simulink model "car_model_FIXED"  (R2022b)
settings: Solver=VariableStepAuto  StartTime=0.0  StopTime=60  RelTol=1e-3
values from neighbouring files (symbols this model uses):
  ABS_MAX_TORQUE = [25 25 25 25]    [workspace.mat]
  ABS_MAX_TRQ_CMD = 50    [workspace.mat]
  ABS_MIN_TORQUE = [0.01 0.01 0.01 0.01]    [workspace.mat]
  acc_IC = 0    [workspace.mat]
  ACCELERATION_MAX = 30    [workspace.mat]
  ActSuspDutyCycle = 1    [workspace.mat]
  Aeq_left = [0.305756190204 0.308857786592 0.311945941182 0.315020811431 0.318082554689 0.321131328186 0.324167289011 0.327190594103 0.330201400225 0.333199863958 0.336186141681 0.339160389558 ... (261 elements, 1x261)]    [workspace.mat]
  Aeq_right = [-0.961664782545 -0.959835898365 -0.957982924115 -0.956106413788 -0.954206913862 -0.952284963337 -0.950341093764 -0.948375829284 -0.946389686656 -0.944383175301 -0.942356797333 -0.940311047601 ... (261 elements, 1x261)]    [workspace.mat]
  alpha_error = 0.1    [workspace.mat]
  ang_acc_hystersesis = 0.1    [workspace.mat]
  ang_IC = 0    [workspace.mat]
  ang_vel_IC = 0    [workspace.mat]
  area_air = 0.15    [workspace.mat]
  axb = -5    [workspace.mat]
  battery_current_IC = 0    [workspace.mat]
  BATTERY_CURRENT_MAX = 140    [workspace.mat]
  BATTERY_CURRENT_MIN = 0    [workspace.mat]
  battery_FT_IC = 300    [workspace.mat]
  battery_T_IC = 300    [workspace.mat]
  BATTERY_TEMPERATURE_MAX = 60    [workspace.mat]
  BATTERY_TEMPERATURE_MIN = 0    [workspace.mat]
  battery_voltage_IC = 332    [workspace.mat]
  BATTERY_VOLTAGE_MAX = 340    [workspace.mat]
  BATTERY_VOLTAGE_MIN = 60    [workspace.mat]
  br = 0.01    [workspace.mat]
  brake_bias = [0.35 0.35 0.15 0.15]    [workspace.mat]
  Brake_Pressure_IC = 1    [workspace.mat]
  ccl_IC = 0    [workspace.mat]
  CENTER_STEER_ANGLE_MAX = 130    [workspace.mat]
  covarience_matrix_IC = [0.001 0 0 0 0 0 0 0 0 0 0 0 ... (784 elements, 28x28)]    [workspace.mat]
  CURRENT_BUFFER = 25    [workspace.mat]
  cy_sweep = [13568.4166816 14020.2069783 14456.754831 14879.7402576 15289.7264712 15687.2766846 16072.954111 16447.3219632 16810.9434544 17164.3817975 17508.2002054 17842.9618912 ... (101 elements, 1x101)]    [workspace.mat]
  dB = 0.001    [workspace.mat]
  dcl_IC = 140    [workspace.mat]
  DCL_MAX = 130    [workspace.mat]
  DCL_MIN = 0    [workspace.mat]
  deadband_angle = 12    [workspace.mat]
  dIndex = 50    [workspace.mat]
  driver_t = 0.015    [workspace.mat]
  dt_OFF = 4.5    [workspace.mat]
  dt_ON = 7.5    [workspace.mat]
  dTx = 0.01    [workspace.mat]
  dx = 0.1    [workspace.mat]
  dZ = 0.295    [workspace.mat]
  efficiency_grid = [0.759500051293 0.787587791453 0.809832189108 0.826747821898 0.837164543102 0.842744381136 0.842258400104 0.838611650621 0.82826195101 0.814029316176 0.795690627225 0.7759791486 ... (2782 elements, 26x107)]    [workspace.mat]
  F0z = [0 0]    [workspace.mat]
  forward_look_straight = 5    [workspace.mat]
  forward_look_turn = 15    [workspace.mat]
  Fz_IC = 539.55    [workspace.mat]
  Fz_sweep = [200 210 220 230 240 250 260 270 280 290 300 310 ... (101 elements, 1x101)]    [workspace.mat]
  g = 9.81    [workspace.mat]
  GAIN_ABS = 100    [workspace.mat]
  gearbox_efficiency = [0.8 0.8 0.8 0.8]    [workspace.mat]
  gps_counter_IC = 0    [workspace.mat]
  gps_hz = 0.01    [workspace.mat]
  gr = [8.74786324786 8.74786324786 8.74786324786 8.74786324786]    [workspace.mat]
  I = 0    [workspace.mat]
  I_Driver = 1    [workspace.mat]
  indicies = [3 3.5 4 0.5 1 1.5 2 2.5 3 3.5 4 0.5 ... (27 elements, 1x27)]    [workspace.mat]
  IYY = 0.3    [workspace.mat]
  kx_sweep = [8779.958 9178.302 9576.646 9974.99 10373.334 10771.678 11170.022 11568.366 11966.71 12365.054 12763.398 13161.742 ... (101 elements, 1x101)]    [workspace.mat]
  l = [0.772 0.772]    [workspace.mat]
  lambda_star = 0.15    [workspace.mat]
  low_V_SA = 0.001    [workspace.mat]
  lr = 35    [workspace.mat]
  m_all = 220    [workspace.mat]
  m_body = 180    [workspace.mat]
  m_unsprung = [6 6 14 14]    [workspace.mat]
  MAG_MAX = 200    [workspace.mat]
  Max_Brake_Pressure = 100000000    [workspace.mat]
  Max_Driver_Input = 1    [workspace.mat]
  MAX_DTHETA_DRIVER = 360    [workspace.mat]
  MAX_I_Driver = 1    [workspace.mat]
  MAX_STEERING_ADJUST = 15    [workspace.mat]
  max_yaw = [0.705271610162 0.928228152446 1.12280857731 1.14131008363 1.08727026041 1.01377803859 0.938114723816 0.8718206875 0.815009168116 0.767481919497 0.727119764215 0.694403589394 ... (15 elements, 1x15)]    [workspace.mat]
  Min_Brake_Pressure = 1    [workspace.mat]
  Min_Driver_Input = 0    [workspace.mat]
  min_velocity_regen = 1.4    [workspace.mat]
  motor_current_IC = 0    [workspace.mat]
  MOTOR_CURRENT_MAX = 70    [workspace.mat]
  MOTOR_CURRENT_MIN = 0    [workspace.mat]
  MOTOR_ENABLE = [0 0 1 1]    [workspace.mat]
  motor_FT_IC = 300    [workspace.mat]
  motor_T_IC = 300    [workspace.mat]
  MOTOR_TEMPERATURE_MAX = 100    [workspace.mat]
  MOTOR_TEMPERATURE_MIN = 0    [workspace.mat]
  motor_voltage_IC = 332    [workspace.mat]
  MOTOR_VOLTAGE_MAX = 340    [workspace.mat]
  MOTOR_VOLTAGE_MIN = 90    [workspace.mat]
  motorControllerCurve = [25  260; 50  130; 75  0]    [workspace.mat]
  motorTempCurve = [140 138.6 134.4 127.4 117.6 105 89.6 71.4 50.4 26.6 0]    [workspace.mat]
  motorTempX = [75 77 79 81 83 85 87 89 91 93 95]    [workspace.mat]
  mu_star = 0.5    [workspace.mat]
  mx_sweep = [3.38348 3.3655067 3.3477908 3.3303323 3.3131312 3.2961875 3.2795012 3.2630723 3.2469008 3.2309867 3.21533 3.1999307 ... (101 elements, 1x101)]    [workspace.mat]
  my_sweep = [3.036232 3.015241699 2.994987032 2.975452753 2.956623616 2.938484375 2.921019784 2.904214597 2.888053568 2.872521451 2.857603 2.843282969 ... (101 elements, 1x101)]    [workspace.mat]
  noise_state = [1e-06 1e-06 1e-06 1e-06 0.005 0.005 0.005 1e-06 1e-06 1e-06 1e-06 1e-06 ... (28 elements, 28x1)]    [workspace.mat]
  omega_IC = 0    [workspace.mat]
  OMEGA_MAX = 150    [workspace.mat]
  OMEGA_MIN = 0    [workspace.mat]
  ORIENTATION_MAX = 360    [workspace.mat]
  P = 2    [workspace.mat]
  P_Driver = 0.7    [workspace.mat]
  P_High_Speed = 0.1    [workspace.mat]
  P_Steering_Adjust = 2    [workspace.mat]
  P_Straight_Adjust = 5    [workspace.mat]
  pos_IC = 0    [workspace.mat]
  POS_MAX = 300    [workspace.mat]
  q_thresh = 0.3    [workspace.mat]
  RE = 0.223    [workspace.mat]
  rho = 1.225    [workspace.mat]
  s = [0.649 0.621]    [workspace.mat]
  selected_maxvm = [49.86390724 16.21289794 8.219813569 8.05215527 7.103352929 8.35634983 13.87515039 8.72402841 22.75224945 36.67909339 19.32001297 25.09036962 ... (63 elements, 21x3)]    [workspace.mat]
  selected_sweep = [3 3 3 3 3 3 3 3 3 3 3 3 ... (1288 elements, 644x2)]    [workspace.mat]
  selected_track = [inf inf inf inf inf inf inf inf inf inf inf inf ... (37971 elements, 4219x9)]    [workspace.mat]
  shock_length_IC = 0.1    [workspace.mat]
  SHOCK_LENGTH_MAX = 0.25    [workspace.mat]
  SHOCK_LENGTH_MIN = 0    [workspace.mat]
  state_IC = [1 0 0 0 0 0 0 0 0 0 0 0 ... (28 elements, 28x1)]    [workspace.mat]
  steering_sweep = [0 5 10 15 20 25 30 35 40 45 50 55 ... (27 elements, 1x27)]    [workspace.mat]
  steering_Up_Grid = [0.551231966244 8.36038106007 16.1333806643 23.9559539118 31.8240691982 39.7561724339 47.7157531433 55.7845698794 64.1341708168 73.0798046026 82.7903081349 93.1297322155 ... (615 elements, 41x15)]    [workspace.mat]
  ... (+25 more)
undefined symbols (not defined in the file or in its folder): ax, ay, az, covA, covG, covM, covP, covV, DiscIntNeverNeededParam, fusion_t, fusion_t_sim, gps_ratio, IMU_accel, IMU_gyro, imu_hz, IMU_mag, location_lla_IC, p, phi, psi, q, r, sus, theta, trn, veh, VEH, whl, X, Xdot, Y, Ydot, Z, Zdot
libraries: fl_lib x82, nesl_utility x32, vehdynlibtire x10, vehdynlibsuspension x8, simulink x5, autolibutils x5, sharedtransform x5, sdl_lib x4, EngineCoolingComponents_lib x4, slpidlib x3, SimscapeFluids_lib x3, shared6dof x2
(part 14 of 14)

== system car_model_FIXED/Vehicle Model/Wheels and Tires/VDBS/Tires/Fiala Tires/z ==
  In1 : Inport
  In2 : Inport  Port=2
  In3 : Inport  Port=3
  In4 : Inport  Port=4
  Bus Selector{,1..3} (4 alike) : BusSelector  OutputSignals=z
  Vector Concatenate : Concatenate  NumInputs=4
  Out1 : Outport  VectorParamsAs1DForOutWhenUnconnected=off
  wires:
  Bus Selector3/1 -> Vector Concatenate/4  "<z>"
  Bus Selector2/1 -> Vector Concatenate/3  "<z>"
  Bus Selector1/1 -> Vector Concatenate/2  "<z>"
  In4/1 -> Bus Selector3/1
  In3/1 -> Bus Selector2/1
  In2/1 -> Bus Selector1/1
  Bus Selector/1 -> Vector Concatenate/1  "<z>"
  In1/1 -> Bus Selector/1
  Vector Concatenate/1 -> Out1/1

== system car_model_FIXED/Vehicle Model/Wheels and Tires/VDBS/Tires/Fiala Tires/zdot ==
  In1 : Inport
  In2 : Inport  Port=2
  In3 : Inport  Port=3
  In4 : Inport  Port=4
  Bus Selector{,1..3} (4 alike) : BusSelector  OutputSignals=zdot
  Vector Concatenate : Concatenate  NumInputs=4
  Out1 : Outport  VectorParamsAs1DForOutWhenUnconnected=off
  wires:
  Vector Concatenate/1 -> Out1/1
  In1/1 -> Bus Selector/1
  Bus Selector/1 -> Vector Concatenate/1  "<zdot>"
  In2/1 -> Bus Selector1/1
  In3/1 -> Bus Selector2/1
  In4/1 -> Bus Selector3/1
  Bus Selector1/1 -> Vector Concatenate/2  "<zdot>"
  Bus Selector2/1 -> Vector Concatenate/3  "<zdot>"
  Bus Selector3/1 -> Vector Concatenate/4  "<zdot>"

== system car_model_FIXED/Vehicle Model/Wheels and Tires/VDBS/Tires/MF Tires/Fx ==
  In1 : Inport
  In2 : Inport  Port=2
  In3 : Inport  Port=3
  In4 : Inport  Port=4
  Bus Selector{,1..3} (4 alike) : BusSelector  OutputSignals=Fx
  Vector Concatenate : Concatenate  NumInputs=4
  Out1 : Outport  VectorParamsAs1DForOutWhenUnconnected=off
  wires:
  Bus Selector3/1 -> Vector Concatenate/4  "<Fx>"
  Bus Selector2/1 -> Vector Concatenate/3  "<Fx>"
  Bus Selector1/1 -> Vector Concatenate/2  "<Fx>"
  In4/1 -> Bus Selector3/1
  In3/1 -> Bus Selector2/1
  In2/1 -> Bus Selector1/1
  Bus Selector/1 -> Vector Concatenate/1  "<Fx>"
  In1/1 -> Bus Selector/1
  Vector Concatenate/1 -> Out1/1

== system car_model_FIXED/Vehicle Model/Wheels and Tires/VDBS/Tires/MF Tires/Fy ==
  In1 : Inport
  In2 : Inport  Port=2
  In3 : Inport  Port=3
  In4 : Inport  Port=4
  Bus Selector{,1..3} (4 alike) : BusSelector  OutputSignals=Fy
  Vector Concatenate : Concatenate  NumInputs=4
  Out1 : Outport  VectorParamsAs1DForOutWhenUnconnected=off
  wires:
  Vector Concatenate/1 -> Out1/1
  In1/1 -> Bus Selector/1
  Bus Selector/1 -> Vector Concatenate/1  "<Fy>"
  In2/1 -> Bus Selector1/1
  In3/1 -> Bus Selector2/1
  In4/1 -> Bus Selector3/1
  Bus Selector1/1 -> Vector Concatenate/2  "<Fy>"
  Bus Selector2/1 -> Vector Concatenate/3  "<Fy>"
  Bus Selector3/1 -> Vector Concatenate/4  "<Fy>"

== system car_model_FIXED/Vehicle Model/Wheels and Tires/VDBS/Tires/MF Tires/Fz ==
  In1 : Inport
  In2 : Inport  Port=2
  In3 : Inport  Port=3
  In4 : Inport  Port=4
  Bus Selector{,1..3} (4 alike) : BusSelector  OutputSignals=Fz
  Vector Concatenate : Concatenate  NumInputs=4
  Out1 : Outport  VectorParamsAs1DForOutWhenUnconnected=off
  wires:
  Vector Concatenate/1 -> Out1/1
  In1/1 -> Bus Selector/1
  Bus Selector/1 -> Vector Concatenate/1  "<Fz>"
  In2/1 -> Bus Selector1/1
  In3/1 -> Bus Selector2/1
  In4/1 -> Bus Selector3/1
  Bus Selector1/1 -> Vector Concatenate/2  "<Fz>"
  Bus Selector2/1 -> Vector Concatenate/3  "<Fz>"
  Bus Selector3/1 -> Vector Concatenate/4  "<Fz>"

== system car_model_FIXED/Vehicle Model/Wheels and Tires/VDBS/Tires/MF Tires/Mx ==
  In1 : Inport
  In2 : Inport  Port=2
  In3 : Inport  Port=3
  In4 : Inport  Port=4
  Bus Selector{,1..3} (4 alike) : BusSelector  OutputSignals=Mx
  Vector Concatenate : Concatenate  NumInputs=4
  Out1 : Outport  VectorParamsAs1DForOutWhenUnconnected=off
  wires:
  Vector Concatenate/1 -> Out1/1
  In1/1 -> Bus Selector/1
  Bus Selector/1 -> Vector Concatenate/1  "<Mx>"
  In2/1 -> Bus Selector1/1
  In3/1 -> Bus Selector2/1
  In4/1 -> Bus Selector3/1
  Bus Selector1/1 -> Vector Concatenate/2  "<Mx>"
  Bus Selector2/1 -> Vector Concatenate/3  "<Mx>"
  Bus Selector3/1 -> Vector Concatenate/4  "<Mx>"

== system car_model_FIXED/Vehicle Model/Wheels and Tires/VDBS/Tires/MF Tires/My ==
  In1 : Inport
  In2 : Inport  Port=2
  In3 : Inport  Port=3
  In4 : Inport  Port=4
  Bus Selector{,1..3} (4 alike) : BusSelector  OutputSignals=My
  Vector Concatenate : Concatenate  NumInputs=4
  Out1 : Outport  VectorParamsAs1DForOutWhenUnconnected=off
  wires:
  Bus Selector3/1 -> Vector Concatenate/4  "<My>"
  Bus Selector2/1 -> Vector Concatenate/3  "<My>"
  Bus Selector1/1 -> Vector Concatenate/2  "<My>"
  In4/1 -> Bus Selector3/1
  In3/1 -> Bus Selector2/1
  In2/1 -> Bus Selector1/1
  Bus Selector/1 -> Vector Concatenate/1  "<My>"
  In1/1 -> Bus Selector/1
  Vector Concatenate/1 -> Out1/1

== system car_model_FIXED/Vehicle Model/Wheels and Tires/VDBS/Tires/MF Tires/Mz ==
  In1 : Inport
  In2 : Inport  Port=2
  In3 : Inport  Port=3
  In4 : Inport  Port=4
  Bus Selector{,1..3} (4 alike) : BusSelector  OutputSignals=Mz
  Vector Concatenate : Concatenate  NumInputs=4
  Out1 : Outport  VectorParamsAs1DForOutWhenUnconnected=off
  wires:
  Bus Selector3/1 -> Vector Concatenate/4  "<Mz>"
  Bus Selector2/1 -> Vector Concatenate/3  "<Mz>"
  Bus Selector1/1 -> Vector Concatenate/2  "<Mz>"
  In4/1 -> Bus Selector3/1
  In3/1 -> Bus Selector2/1
  In2/1 -> Bus Selector1/1
  Bus Selector/1 -> Vector Concatenate/1  "<Mz>"
  In1/1 -> Bus Selector/1
  Vector Concatenate/1 -> Out1/1

== system car_model_FIXED/Vehicle Model/Wheels and Tires/VDBS/Tires/MF Tires/Re ==
  In1 : Inport
  In2 : Inport  Port=2
  In3 : Inport  Port=3
  In4 : Inport  Port=4
  Bus Selector{,1..3} (4 alike) : BusSelector  OutputSignals=Re
  Vector Concatenate : Concatenate  NumInputs=4
  Out1 : Outport  VectorParamsAs1DForOutWhenUnconnected=off
  wires:
  Vector Concatenate/1 -> Out1/1
  In1/1 -> Bus Selector/1
  Bus Selector/1 -> Vector Concatenate/1  "<Re>"
  In2/1 -> Bus Selector1/1
  In3/1 -> Bus Selector2/1
  In4/1 -> Bus Selector3/1
  Bus Selector1/1 -> Vector Concatenate/2  "<Re>"
  Bus Selector2/1 -> Vector Concatenate/3  "<Re>"
  Bus Selector3/1 -> Vector Concatenate/4  "<Re>"

== system car_model_FIXED/Vehicle Model/Wheels and Tires/VDBS/Tires/MF Tires/alpha ==
  In1 : Inport
  In2 : Inport  Port=2
  In3 : Inport  Port=3
  In4 : Inport  Port=4
  Bus Selector{,1..3} (4 alike) : BusSelector  OutputSignals=Alpha
  Vector Concatenate : Concatenate  NumInputs=4
  Out1 : Outport  VectorParamsAs1DForOutWhenUnconnected=off
  wires:
  Vector Concatenate/1 -> Out1/1
  In1/1 -> Bus Selector/1
  Bus Selector/1 -> Vector Concatenate/1  "<Alpha>"
  In2/1 -> Bus Selector1/1
  In3/1 -> Bus Selector2/1
  In4/1 -> Bus Selector3/1
  Bus Selector1/1 -> Vector Concatenate/2  "<Alpha>"
  Bus Selector2/1 -> Vector Concatenate/3  "<Alpha>"
  Bus Selector3/1 -> Vector Concatenate/4  "<Alpha>"

== system car_model_FIXED/Vehicle Model/Wheels and Tires/VDBS/Tires/MF Tires/kappa ==
  In1 : Inport
  In2 : Inport  Port=2
  In3 : Inport  Port=3
  In4 : Inport  Port=4
  Bus Selector{,1..3} (4 alike) : BusSelector  OutputSignals=Kappa
  Vector Concatenate : Concatenate  NumInputs=4
  Out1 : Outport  VectorParamsAs1DForOutWhenUnconnected=off
  wires:
  Bus Selector3/1 -> Vector Concatenate/4  "<Kappa>"
  Bus Selector2/1 -> Vector Concatenate/3  "<Kappa>"
  Bus Selector1/1 -> Vector Concatenate/2  "<Kappa>"
  In4/1 -> Bus Selector3/1
  In3/1 -> Bus Selector2/1
  In2/1 -> Bus Selector1/1
  Bus Selector/1 -> Vector Concatenate/1  "<Kappa>"
  In1/1 -> Bus Selector/1
  Vector Concatenate/1 -> Out1/1

== system car_model_FIXED/Vehicle Model/Wheels and Tires/VDBS/Tires/MF Tires/omega ==
  In1 : Inport
  In2 : Inport  Port=2
  In3 : Inport  Port=3
  In4 : Inport  Port=4
  Bus Selector{,1..3} (4 alike) : BusSelector  OutputSignals=Omega
  Vector Concatenate : Concatenate  NumInputs=4
  Out1 : Outport  VectorParamsAs1DForOutWhenUnconnected=off
  wires:
  In1/1 -> Bus Selector/1
  Bus Selector/1 -> Vector Concatenate/1  "<Omega>"
  In2/1 -> Bus Selector1/1
  In3/1 -> Bus Selector2/1
  In4/1 -> Bus Selector3/1
  Bus Selector1/1 -> Vector Concatenate/2  "<Omega>"
  Bus Selector2/1 -> Vector Concatenate/3  "<Omega>"
  Bus Selector3/1 -> Vector Concatenate/4  "<Omega>"
  Vector Concatenate/1 -> Out1/1

== system car_model_FIXED/Vehicle Model/Wheels and Tires/VDBS/Tires/MF Tires/z ==
  In1 : Inport
  In2 : Inport  Port=2
  In3 : Inport  Port=3
  In4 : Inport  Port=4
  Bus Selector{,1..3} (4 alike) : BusSelector  OutputSignals=z
  Vector Concatenate : Concatenate  NumInputs=4
  Out1 : Outport  VectorParamsAs1DForOutWhenUnconnected=off
  wires:
  Bus Selector3/1 -> Vector Concatenate/4  "<z>"
  Bus Selector2/1 -> Vector Concatenate/3  "<z>"
  Bus Selector1/1 -> Vector Concatenate/2  "<z>"
  In4/1 -> Bus Selector3/1
  In3/1 -> Bus Selector2/1
  In2/1 -> Bus Selector1/1
  Bus Selector/1 -> Vector Concatenate/1  "<z>"
  In1/1 -> Bus Selector/1
  Vector Concatenate/1 -> Out1/1

== system car_model_FIXED/Vehicle Model/Wheels and Tires/VDBS/Tires/MF Tires/zdot ==
  In1 : Inport
  In2 : Inport  Port=2
  In3 : Inport  Port=3
  In4 : Inport  Port=4
  Bus Selector{,1..3} (4 alike) : BusSelector  OutputSignals=zdot
  Vector Concatenate : Concatenate  NumInputs=4
  Out1 : Outport  VectorParamsAs1DForOutWhenUnconnected=off
  wires:
  Vector Concatenate/1 -> Out1/1
  In1/1 -> Bus Selector/1
  Bus Selector/1 -> Vector Concatenate/1  "<zdot>"
  In2/1 -> Bus Selector1/1
  In3/1 -> Bus Selector2/1
  In4/1 -> Bus Selector3/1
  Bus Selector1/1 -> Vector Concatenate/2  "<zdot>"
  Bus Selector2/1 -> Vector Concatenate/3  "<zdot>"
  Bus Selector3/1 -> Vector Concatenate/4  "<zdot>"

== matlab function car_model_FIXED/Vehicle Model/Vehicle/6DOF/Suspension to Chasiss Transforms/Estimated Unsprung Mass Orientation ==
  data: angles output size=3; angleIn input size=3; GeomXYZ output size=3; GemoXYZIn input size=3; Ground input size=4; trackW parameter; wheelB parameter
function [angles,GeomXYZ]= three26(angleIn, GemoXYZIn, Ground,trackW, wheelB)%#codegen
coder.allowpcode('plain')
% Copyright 2018 The MathWorks, Inc.
[angles,GeomXYZ]= vdynthree2six(angleIn, GemoXYZIn, Ground,trackW, wheelB);

== matlab function car_model_FIXED/Driver & Environment/Reference Generator/Reference Geneator ==
  data: index_small input; index_all input; psi input; deg2rad parameter; Vg input; yaw input; pos input; omega input; index_small output; index_all output; v_error output; d_error output; psi_error output; v_cog output; r_ref output; r_error output; x_ref output; y_ref output; yaw_ref output; omega output; p_error output; Vnow output; ahead output; ahead input; selected_track parameter; dIndex parameter; dx parameter; forward_look_straight parameter; forward_look_turn parameter; q_thresh parameter; indicies parameter; selected_maxvm parameter; axb parameter; di_now output; di_prev input
function [index_small, index_all, v_error, d_error, psi_error, v_cog, r_ref, r_error, x_ref, y_ref, yaw_ref, omega, p_error,Vnow, ahead, di_now] = ref_gen(index_small, index_all, psi, deg2rad, Vg, yaw, pos, omega, ahead, selected_track, dIndex, dx, forward_look_straight, forward_look_turn, q_thresh, indicies, selected_maxvm, axb, di_prev)
%% Extract Data
Y_all = selected_track(index_all:index_all+dIndex,2);
X_all = selected_track(index_all:index_all+dIndex,3);

Vmax_now = selected_maxvm(index_small,3);
num_elem = length(selected_maxvm(:,1));

if num_elem > index_small
    Vmax_next = selected_maxvm(index_small+1,3);
    d_next = selected_maxvm(index_small+1,1);
else
    Vmax_next = Vmax_now;
    d_next = 100;
end

%% Determine Reference Point
d_error_all = sqrt((Y_all - pos.Y).^2 + (X_all - pos.X).^2);
[min_d, min_index] = min(d_error_all);
index_all = index_all + min_index - 1;

%% Aquire Reference Values
y_ref = selected_track(index_all, 2);
x_ref = selected_track(index_all, 3);
y_ref_next = selected_track(index_all+5, 2);
x_ref_next = selected_track(index_all+5, 3);
r_ref = selected_track(index_all, 4);
r_straight = selected_track(index_all+forward_look_straight, 4);
r_turn = selected_track(index_all+forward_look_turn, 4);
turn_ref = selected_track(index_all, 5);
straight_next = selected_track(index_all+forward_look_straight, 5);
turn_next = selected_track(index_all+forward_look_turn, 5);
psi_ref = selected_track(index_all, 8);
di_now = selected_track(index_all, 9);

%% Velocity Error
v_cog = sqrt((Vg.xdot^2) + (Vg.ydot^2));

if ahead
    di = (di_now*dx) + d_next;
else
    di = di_now*dx;
end

det = v_cog^2 + (2*axb*di);

if det < 0
    Vnext = 0;
else
    Vnext = sqrt(det);
end

increment = 0;

if (abs(Vmax_next - Vnext) < 0.25) && (Vmax_now > Vmax_next) && (~ahead)
    Vnow = Vmax_next;
    index_small = index_small + 1;
    ahead = 1;
    increment = 1;
elseif ((di_now - di_prev) > 0) && ~ahead
    Vnow = Vmax_next;
    index_small = index_small + 1;
else
    Vnow = Vmax_now;
end

if ((di_now - di_prev) > 0) && ~increment
    ahead = 0;
end

% if r_ref ~= inf
%     Vnow = min(Vnow, 17);
% end

v_error = Vnow - v_cog - 1;

%% Turning Radius Error
if (turn_ref ~= straight_next) || (r_ref ~= r_straight)
    turn_ref = straight_next;
    r_ref = r_straight;
elseif (turn_ref ~= turn_next) && (turn_next ~= 0) && (turn_ref ~= 0)
    turn_ref = turn_next;
    r_ref = r_turn;
end

r_IC = abs(v_cog / yaw);
r_error = turn_ref *  ((1 / r_ref) - (1 / r_IC));

if r_ref == inf
    yaw_ref = 0;
else
    yaw_ref = turn_ref * v_cog / r_ref;
end

%% Angle Error
sign_steer = 1;

if (abs(psi - psi_ref) > pi) && (sign(psi) ~= sign(psi_ref))
    if psi < 0
        sign_steer = -1;
    end
elseif (psi > psi_ref)
    sign_steer = -1;   
end

if abs(psi_ref - psi) < pi
    psi_error = sign_steer * abs(psi_ref - psi) / deg2rad;
else
    psi_error = sign_steer * ((pi - abs(psi_ref)) + (pi - abs(psi))) / deg2rad;
end

%% Distance Error
% Determine Vehicle Quadrant
if (pos.Y - y_ref) > q_thresh
   if (pos.X - x_ref) > q_thresh
       Qc = 5;
   elseif (pos.X - x_ref) < -q_thresh
       Qc = 11;
   else
       Qc = 4;
   end
elseif (pos.Y - y_ref) < -q_thresh
   if (pos.X - x_ref) > q_thresh
       Qc = 7;
   elseif (pos.X - x_ref) < -q_thresh
       Qc = 9;
   else
       Qc = 8;
   end
else
   if (pos.X - x_ref) > q_thresh
       Qc = 6;
   elseif (pos.X - x_ref) < -q_thresh
       Qc = 10;
   else
       Qc = 0;
   end
end

% Determine Next Reference Point Quadrant
if y_ref_next > y_ref
   if x_ref_next > x_ref
       Qn = 5;
   elseif x_ref_next < x_ref
       Qn = 11;
   else
       Qn = 4;
   end
elseif y_ref_next < y_ref
   if x_ref_next > x_ref
       Qn = 7;
   elseif x_ref_next < x_ref
       Qn = 9;
   else
       Qn = 8;
   end
else
   if x_ref_next > x_ref
       Qn = 6;
   elseif x_ref_next < x_ref
       Qn = 10;
   else
       Qn = 0;
   end
end

% Determine Sign for Distance Error
if Qc == 0
   sign_distance = 0;
elseif (abs(x_ref_next - x_ref) == abs(pos.X - x_ref)) && (abs(y_ref_next - y_ref) == abs(pos.Y - y_ref))
   sign_distance = 0;
elseif ((Qc ~= Qn) && (indicies(Qc+4) ~= Qn))
    if (indicies(Qc+1) == indicies(Qn)) || (indicies(Qc+2) == indicies(Qn)) || (indicies(Qc+3) == indicies(Qn))
        sign_distance = -1;
    else
        sign_distance = 1;
    end
else
    if indicies(Qc) == 1 || indicies(Qc) == 3
        y_axis = y_ref;
    elseif indicies(Qc) == 4
        y_axis = y_ref + 1;
    else
        y_axis = y_ref - 1;
    end
    
    if indicies(Qc) == 2 || indicies(Qc) == 4
        x_axis = x_ref;
    elseif indicies(Qc) == 1
        x_axis = x_ref + 1;
    else
        x_axis = x_ref - 1;
    end
    
    axis_coordiantes = [y_axis, x_axis];
    ref_coordiantes = [y_ref, x_ref];
    next_ref_coordinates = [y_ref_next, x_ref_next];
    vehicle_coordinates = [pos.Y, pos.X];
    
    ref_vec = axis_coordiantes - ref_coordiantes;
    veh_vec = vehicle_coordinates - ref_coordiantes;
    next_ref = next_ref_coordinates - ref_coordiantes;
    
    theta_veh_ref = acos(dot(ref_vec, veh_vec) / (norm(ref_vec)*norm(veh_vec)));
    theta_next_ref = acos(dot(ref_vec, next_ref) / (norm(ref_vec)*norm(next_ref)));
    
    if theta_veh_ref < theta_next_ref
        sign_distance = 1;
    else
        sign_distance = -1;
    end
end

d_error = sign_distance * min_d;

%% Combined Purtubation Error
if (sign_distance~=sign(psi_error)) && (d_error~=0)
    p_error = d_error;
else
    p_error = psi_error;
end

end

== matlab function car_model_FIXED/Driver & Environment/Longitudinal Control/ABS/ABS system/MATLAB Function1 ==
  data: u input; y output; mu_star parameter; lambda_star parameter
function y = fcn(u,mu_star, lambda_star)

    y = (2.*mu_star.*lambda_star.*u./(lambda_star.^2+u.^2));

end

== matlab function car_model_FIXED/Driver & Environment/Sweep Generator/Sweep Generator ==
  data: index input; index output; vel input; ON input; vel_err output; ref_steer output; ON output; selected_sweep parameter; dt_ON parameter; dt_OFF parameter; counter output; counter input; tvs_t_sim parameter
function [index, vel_err,ref_steer, ON, counter] = fcn(index, vel, ON, selected_sweep, dt_ON, dt_OFF, counter, tvs_t_sim)

% Update Control Output
ref_vel = selected_sweep(index, 1);
ref_steer = selected_sweep(index, 2);
vel_err = ref_vel - norm([vel.xdot vel.ydot]);
counter = counter + 1;

% Update Scenario
if ((counter*tvs_t_sim) == dt_ON && ON) || ((counter*tvs_t_sim) == dt_OFF && ~ON)
    index = index + 1;
    counter = 0;

    if (selected_sweep(index, 2) == 0 && index > 1)
        ON = double(~ON);
    end

end

== matlab function car_model_FIXED/Vehicle Model/Vehicle/6DOF/Suspension to Chasiss Transforms/MATLAB Function ==
  data: u input; y output; aero_coeff parameter
function y = fcn(u, aero_coeff)

Fz = aero_coeff*u^2;


y = [0 0 Fz];

== matlab function car_model_FIXED/Vehicle Model/Electronics/Navigation Sensors/VNED to SNED ==
  data: accel_SNED output; gyro_SNED output; accel_VNED input size=[3 1]; gyro_VNED input size=[3 1]; mag_VNED input size=[3 1]; mag_SNED output; phi parameter
function [accel_SNED, gyro_SNED, mag_SNED] = VNED2SNED(accel_VNED, gyro_VNED, mag_VNED, phi)
%% Define Rotation
IMUNED2VNED = rotmat(quaternion([0 (phi - 180) 0],"eulerd","XYZ","frame"),"frame");
MAGNED2VNED = rotmat(quaternion([180 (180 - phi) 0],"eulerd","XYZ","frame"),"frame");

%% Coordinate Transformation
accel_SNED = IMUNED2VNED\accel_VNED;
gyro_SNED = IMUNED2VNED\gyro_VNED;
mag_SNED = MAGNED2VNED\mag_VNED;

end

== matlab function car_model_FIXED/Vehicle Model/Electronics/Navigation Sensors/integrate angvel ==
  data: Orientation_e input; Orientation_c output; Orientation_e output
function [Orientation_c, Orientation_e]  = fcn(Orientation_e)

Orientation_q = quaternion(Orientation_e, 'euler', 'XYZ', 'frame');

Orientation_c = compact(Orientation_q);

end

== matlab function car_model_FIXED/Control Systems/Sensor Fusion/fusion ==
  data: count input [0..gps_ratio]; count output [0..gps_ratio]; rot_map output [-4..4]; velocity input size=[1,3] [-VELOCITY_MAX..VELOCITY_MAX]; state_out output; position input size=[1,3] [-POS_MAX..POS_MAX]; acceleration input size=[1,3] [-ACCELERATION_MAX..ACCELERATION_MAX]; angularVelocity input size=[1,3] [-YAW_MAX..YAW_MAX]; magField input size=[1,3] [-MAG_MAX..MAG_MAX]; state_in input; cov_in input; covG parameter; covA parameter; covM parameter; covP parameter; covV parameter; fusion_t parameter; location_lla_IC parameter; cov_out output; noise_state parameter; gps_ratio parameter
function [count, rot_map, state_out, cov_out] = fusion(count, velocity, position ,acceleration,angularVelocity, magField, state_in, cov_in, covG, covA, covM, covP, covV, fusion_t, location_lla_IC, noise_state, gps_ratio) 
%% Create Filter
filter = insfilterAsync();
filter.ReferenceLocation = location_lla_IC;
filter.State = state_in;
filter.StateCovariance = cov_in;

filter.QuaternionNoise = noise_state(1:4);
filter.AngularVelocityNoise = noise_state(5:7);
filter.PositionNoise = noise_state(8:10);
filter.VelocityNoise = noise_state(11:13);
filter.AccelerationNoise = noise_state(14:16);
filter.GyroscopeBiasNoise = noise_state(17:19);
filter.AccelerometerBiasNoise = noise_state(20:22);
filter.GeomagneticVectorNoise = noise_state(23:25);
filter.MagnetometerBiasNoise = noise_state(26:28);

%% Sensor Fusion
predict(filter, fusion_t);

fuseaccel(filter,acceleration,covA);
fusegyro(filter,angularVelocity,covG);
fusemag(filter, magField,covM);

if ~count
    fusegps(filter,position,covP,velocity,covV);
end

count = mod(count + 1, gps_ratio);

[~,rot_map,~] = pose(filter, 'rotmat');

%% Save Fusion State & State Covariance
state_out = filter.State;
cov_out = filter.StateCovariance;

end

== matlab function car_model_FIXED/Control Systems/Sensor Fusion/NED2VNED ==
  data: rot_map input [-4..4]; state input; ang output [-1..1]; angvel output [-YAW_MAX..YAW_MAX]; pos output [-POS_MAX..POS_MAX]; vel output [-VELOCITY_MAX..VELOCITY_MAX]; accel output [-ACCELERATION_MAX..ACCELERATION_MAX]; mag output [-MAG_MAX..MAG_MAX]; accel_bias output [-ACCELERATION_MAX..ACCELERATION_MAX]; gyro_bias output [-YAW_MAX..YAW_MAX]; mag_bias output [-MAG_MAX..MAG_MAX]
function [ang,angvel,pos,vel,accel,mag,accel_bias,gyro_bias,mag_bias] = NED2VNED(rot_map, state)
%% Vehicle POSE
ang = state(1:4);                    % quaternion (VNED2SNED)
angvel = state(5:7);                 % chassis angular velocity (rad/s)(VNED)
pos = state(8:10);                   % chassis position (m)(NED)
vel = rot_map*state(11:13);          % chassis velocity (m/s)(VNED)
accel = rot_map*state(14:16);        % chassis acceleration (m/s^2)(VNED)
mag = state(23:25);                  % magnetic field (uT)(NED)

%% Sensor Parameters
accel_bias = rot_map*state(17:19);   % accelerometer bias (m/s^2)(VNED)
gyro_bias = rot_map*state(20:22);    % gyroscope bias (rad/s)(VNED)
mag_bias = state(26:28);             % magnetometer bias (uT)(NED)

end

== matlab function car_model_FIXED/Control Systems/Sensor Fusion/SNED to VNED ==
  data: accel_VNED output size=[3 1] [-ACCELERATION_MAX..ACCELERATION_MAX]; gyro_VNED output size=[3 1] [-YAW_MAX..YAW_MAX]; accel_SNED input [-ACCELERATION_MAX..ACCELERATION_MAX]; gyro_SNED input [-YAW_MAX..YAW_MAX]; mag_SNED input [-MAG_MAX..MAG_MAX]; mag_VNED output size=[3 1] [-MAG_MAX..MAG_MAX]; phi parameter
function [accel_VNED, gyro_VNED, mag_VNED] = SNED2VNED(accel_SNED, gyro_SNED, mag_SNED, phi)
%% Define Rotation
IMUNED2VNED = rotmat(quaternion([0 (phi - 180) 0],"eulerd","XYZ","frame"),"frame");
MAGNED2VNED = rotmat(quaternion([180 (180 - phi) 0],"eulerd","XYZ","frame"),"frame");

%% Coordinate Transformation
accel_VNED = IMUNED2VNED*accel_SNED;  % chassis acceleration (m/s^2)(NED)
gyro_VNED = IMUNED2VNED*gyro_SNED;    % chassis angular velocity (rad/s)(VNED)
mag_VNED = MAGNED2VNED*mag_SNED;      % magnetic field (uT)(NED)

end

== matlab function car_model_FIXED/Driver & Environment/Longitudinal Control/ABS/ABS system/MATLAB Function ==
  data: w_fake input; w input size=[1 4]; v input; tau output; lambda0 input size=[1 4]; vdot input; lambda input size=[1 4]; m_all parameter; RE parameter; IYY parameter; br parameter; d output
function [tau, d]  = fcn(w_fake,w,v,lambda0,vdot,lambda,m_all,RE,IYY,br)

if v > 0
    t1 = -IYY*v./RE.*(lambda-lambda0);
    t2 = -IYY.*w_fake./v.*vdot;
    t3 = -br.*w_fake;
    t4 = -(m_all.*RE.*vdot/4);
    tau = -IYY*v./RE.*(lambda-lambda0)-br.*w_fake-IYY.*w_fake./v.*vdot-(m_all.*RE.*vdot/4);
else
    tau = [0 0 0 0];
    t1 = [0 0 0 0];
    t2 = [0 0 0 0];
    t3 = [0 0 0 0];
    t4 = 0;
end

d1 = sqrt(abs((w(1)^2 - w(3)^2)/w(1)^2));
d2 = sqrt(abs((w(2)^2 - w(4)^2)/w(2)^2));

d = (min(max(d1, d2), 1));

if (w(3) < 3)
    d = 1;
elseif d > 0.5
    d = 0.5;
else
    d = 1;
end
